simulink model "SerialCommunication_OneWay"  (Simulink 8.1)
settings: Solver=ode3  StartTime=0.0  StopTime=30  FixedStep=0.001  RelTol=1e-3
libraries: xpclib x4, GisooLib x1, simulink x1, GisooLib1 x1
settings Model: Creator=behdad  LastModifiedBy=behdad
settings DataIOCC: SignalLoggingSaveFormat=Dataset
settings OptimizationCC: ExpressionDepthLimit=128
settings DebuggingCC: FcnCallInpInsideContextMsg=EnableAllAsError
settings GRTTargetCC: CombineOutputUpdateFcns=on  GRTInterface=off

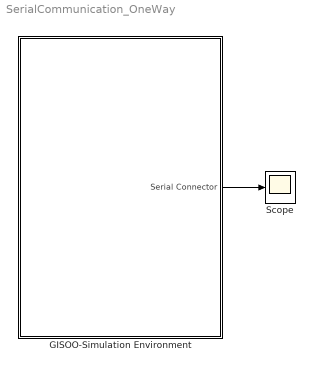
== system SerialCommunication_OneWay ==
  GISOO-Simulation Environment : Subsystem  AncestorBlock=GisooLib/GISOO-Simulation Environment  TreatAsAtomicUnit=on
  Scope : Scope
  wires:
  GISOO-Simulation Environment/1(Serial Connector) -> Scope/1

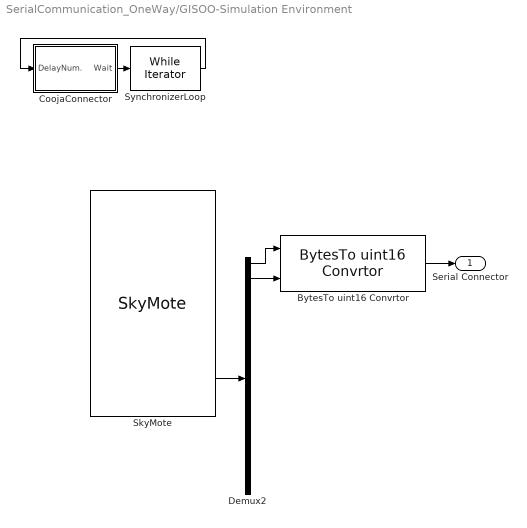
== system SerialCommunication_OneWay/GISOO-Simulation Environment ==
  BytesTo uint16 Convrtor : GisooLib/BytesTo uint16 Convrtor
  CoojaConnector : Subsystem
  Demux2 : Demux  Outputs=16
  SkyMote : GisooLib1/SkyMote  moteID=1  PacketType=6
  SynchronizerLoop : WhileIterator  MaxIters=-1  WhileBlockType=do-while  ShowIterationPort=on
  Serial Connector : Outport
  wires:
  SynchronizerLoop/1 -> CoojaConnector/1(DelayNum.)
  CoojaConnector/1(Wait) -> SynchronizerLoop/1
  SkyMote/3 -> Demux2/1
  Demux2/1 -> BytesTo uint16 Convrtor/1
  Demux2/2 -> BytesTo uint16 Convrtor/2
  BytesTo uint16 Convrtor/1 -> Serial Connector/1

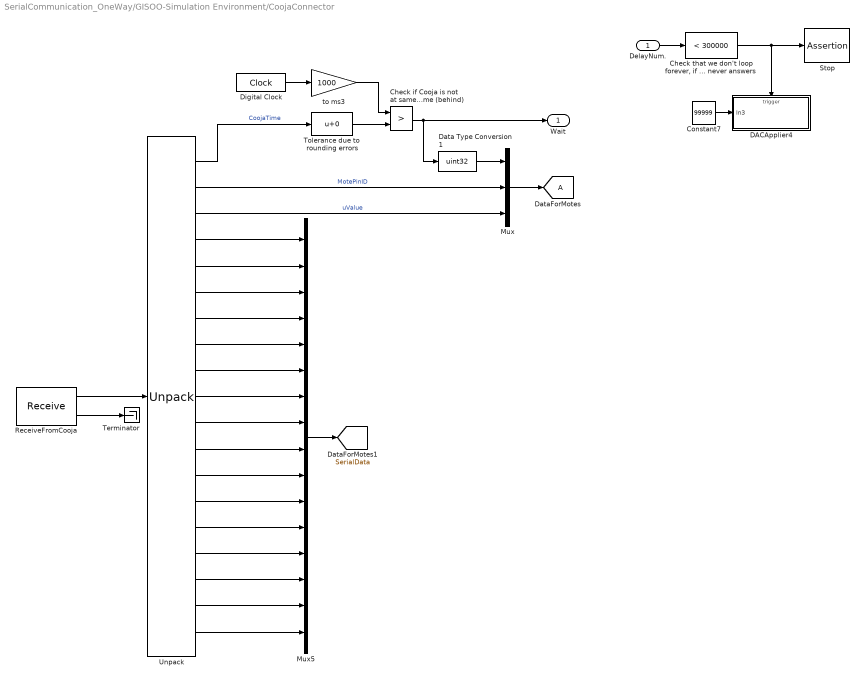
== system SerialCommunication_OneWay/GISOO-Simulation Environment/CoojaConnector ==
  DelayNum. : Inport
  Check if Cooja is not at same time (behind) : RelationalOperator  Operator=>  OutDataTypeStr=boolean
  "Check that we don't loop forever, if Cooja never answers" : simulink/Logic and Bit Operations/Compare To Constant  relop=<  const=300000  OutDataTypeStr=uint8  ZeroCross=off
  Constant7 : Constant  Value=99999
  DACApplier4 : Subsystem  AncestorBlock=BehdadLib/SIm_Cooj Synchronizer/Send  TreatAsAtomicUnit=on
  Data Type Conversion1 : DataTypeConversion  OutDataTypeStr=uint32
  Digital Clock : DigitalClock  SampleTime=-1
  Mux : Mux  Inputs=3
  Mux5 : Mux  Inputs=16
  ReceiveFromCooja : xpclib/UDP/Receive  ipAddress=127.0.0.1  ipPort=55555  width=28  vblLen=off  sampletime=-1
  Stop : Assertion  AssertionFailFcn=warning('No time-synchronization with ns-2');
  Terminator : Terminator
  Tolerance due to rounding errors : Bias
  Unpack : xpclib/UDP/Unpack  dimensions={[1],[1],[1],[1],[1],[1],[1],[1],[1],[1],[1],[1],[1],[1],[1],[1],[1],[1],[1]}  datatypes={'uint32','uint32','uint32','uint8','uint8','uint8','uint8','uint8','uint8','uint8','uint8','uint8','uint8','uint8','uint8','uint8','uint8','uint8','uint8'}  byteAlign=1
  to ms3 : Gain  Gain=1000  ParamDataTypeStr=uint32  OutDataTypeStr=Inherit: Inherit via back propagation
  Wait : Outport
  tag scope: A=global, SerialData=global
  wires:
  Unpack/19 -> Mux5/16
  Unpack/18 -> Mux5/15
  Unpack/17 -> Mux5/14
  Unpack/16 -> Mux5/13
  Unpack/15 -> Mux5/12
  Unpack/14 -> Mux5/11
  Unpack/13 -> Mux5/10
  Unpack/12 -> Mux5/9
  Unpack/11 -> Mux5/8
  Unpack/10 -> Mux5/7
  Unpack/9 -> Mux5/6
  Unpack/8 -> Mux5/5
  Unpack/7 -> Mux5/4
  Unpack/6 -> Mux5/3
  Unpack/5 -> Mux5/2
  Unpack/4 -> Mux5/1
  Mux5/1 -> [SerialData]
  Constant7/1 -> DACApplier4/1(In3)
  Mux/1 -> [A]
  DelayNum./1 -> "Check that we don't loop forever, if Cooja never answers"/1
  "Check that we don't loop forever, if Cooja never answers"/1 -> DACApplier4/Trigger, Stop/1
  Data Type Conversion1/1 -> Mux/1
  Unpack/3 -> Mux/3  "uValue"
  Tolerance due to rounding errors/1 -> Check if Cooja is not at same time (behind)/2
  Digital Clock/1 -> to ms3/1
  ReceiveFromCooja/1 -> Unpack/1
  to ms3/1 -> Check if Cooja is not at same time (behind)/1
  Check if Cooja is not at same time (behind)/1 -> Wait/1, Data Type Conversion1/1
  ReceiveFromCooja/2 -> Terminator/1
  Unpack/1 -> Tolerance due to rounding errors/1  "CoojaTime"
  Unpack/2 -> Mux/2  "MotePinID"

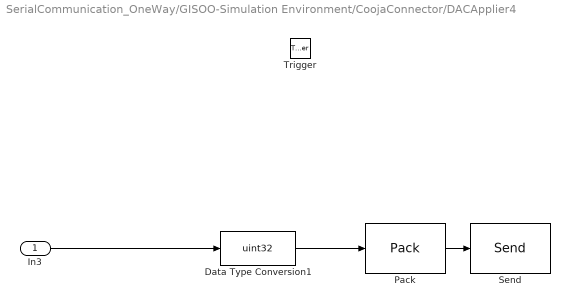
== system SerialCommunication_OneWay/GISOO-Simulation Environment/CoojaConnector/DACApplier4 ==
  In3 : Inport
  Trigger : TriggerPort
  Data Type Conversion1 : DataTypeConversion  OutDataTypeStr=uint32
  Pack : xpclib/UDP/Pack  datatypes={'uint32'}  byteAlign=1
  Send : xpclib/UDP/Send  ipAddress=255.255.255.255  ipPort=18006  localPort=-1  vblLen=off  sampletime=-1
  wires:
  Pack/1 -> Send/1
  Data Type Conversion1/1 -> Pack/1
  In3/1 -> Data Type Conversion1/1
